simulink model "Comunicacion_Telegram_5"  (R2020b)
settings: Solver=FixedStepDiscrete  StartTime=0.0  StopTime=inf  FixedStep=0.01  RelTol=1e-3
libraries: arduinolib x15, simulink x5, pid_lib x2, commutil2 x1
settings Model: SILPILModeSetting=veronly  ExtModeTrigDuration=2  Creator=manol  LastModifiedBy=manol
settings SolverCC: AutoInsertRateTranBlk=on
settings OptimizationCC: EnhancedBackFolding=on  PassReuseOutputArgsAs=Individual arguments  ZeroExternalMemoryAtStartup=off  ZeroInternalMemoryAtStartup=off  MaxStackSize=64  OptimizeBlockOrder=speed  DifferentSizesBufferReuse=on  OptimizationCustomize=off  EfficientTunableParamExpr=on
settings DebuggingCC: ParameterTunabilityLossMsg=error
settings HardwareCC: ProdBitPerInt=16  ProdBitPerPointer=16  ProdBitPerSizeT=16  ProdBitPerPtrDiffT=16  ProdLargestAtomicFloat=None  ProdWordSize=8  ProdHWDeviceType=Atmel->AVR
settings SFSimCC: MATLABDynamicMemAlloc=off
settings RTWCC: Description=Embedded Coder  SystemTargetFile=ert.tlc  HardwareBoard=Arduino Mega 2560  TemplateMakefile=ert_default_tmf  Toolchain=Arduino AVR  BuildConfiguration=Faster Runs
settings CodeAppCC: ForceParamTrailComments=on  IgnoreCustomStorageClasses=off  OperatorAnnotations=on  SimulinkDataObjDesc=on  SFDataObjDesc=on  InsertBlockDesc=on
settings ERTTargetCC: SupportContinuousTime=on  SupportVariableSizeSignals=on  ExtModeStaticAllocSize=2048

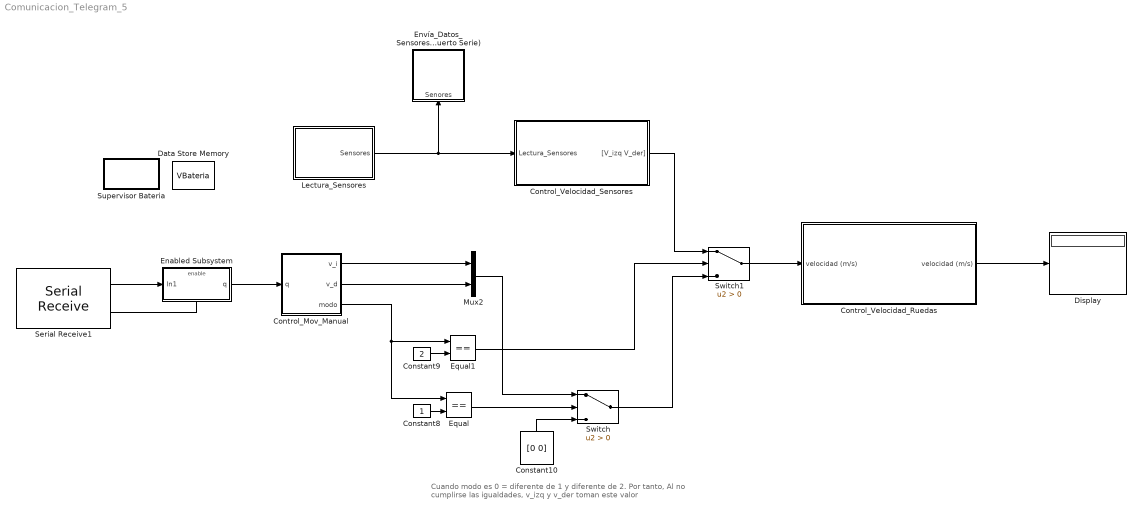
== system Comunicacion_Telegram_5 ==
  note: Cuando modo es 0 = diferente de 1 y diferente de 2.
      | Por tanto, Al no cumplirse las igualdades, v_izq y v_der toman este valor
  Constant10 : Constant  Value=[0 0]
  Constant8 : Constant
  Constant9 : Constant  Value=2
  Control_Mov_Manual : Stateflow chart  TreatAsAtomicUnit=on
  Control_Velocidad_Ruedas : Subsystem
  Control_Velocidad_Sensores : Subsystem
  Data Store Memory : DataStoreMemory  DataStoreName=VBateria  ReadBeforeWriteMsg=warning  WriteAfterWriteMsg=warning  WriteAfterReadMsg=warning  ShowAdditionalParam=off
  Display : Display
  Enabled Subsystem : Subsystem  TreatAsAtomicUnit=on
  Envía_Datos_Sensores (Puerto Serie) : Subsystem
  Equal : RelationalOperator  Operator===  OutDataTypeStr=boolean  RndMeth=Simplest
  Equal1 : RelationalOperator  Operator===  OutDataTypeStr=boolean  RndMeth=Simplest
  Lectura_Sensores : Subsystem
  Mux2 : Mux  Inputs=2
  Serial Receive1 : arduinolib/Serial Receive  isARMArch=off  portNumber=3  DataType=uint8  Datalength=1  SampleTime=0.01  showOutStatus=on  blockPlatform=arduino
      settings: SourceProductBaseCode=ARDUINO
  Supervisor Bateria : Subsystem
  Switch : Switch  Criteria=u2 > Threshold
  Switch1 : Switch  Criteria=u2 > Threshold
  wires:
  Control_Mov_Manual/3(modo) -> Equal/1, Equal1/1
  Constant10/1 -> Switch/3
  Equal1/1 -> Switch1/2
  Constant9/1 -> Equal1/2
  Switch/1 -> Switch1/3
  Serial Receive1/2 -> Enabled Subsystem/Enable
  Control_Mov_Manual/2(v_d) -> Mux2/2
  Constant8/1 -> Equal/2
  Equal/1 -> Switch/2
  Control_Mov_Manual/1(v_i) -> Mux2/1
  Enabled Subsystem/1(q) -> Control_Mov_Manual/1(q)
  Mux2/1 -> Switch/1
  Serial Receive1/1 -> Enabled Subsystem/1(In1)
  Switch1/1 -> Control_Velocidad_Ruedas/1(velocidad (m/s))
  Lectura_Sensores/1(Sensores) -> Control_Velocidad_Sensores/1(Lectura_Sensores), Envía_Datos_Sensores (Puerto Serie)/1(Senores)
  Control_Velocidad_Sensores/1("[V_izq V_der]") -> Switch1/1
  Control_Velocidad_Ruedas/1(velocidad (m/s)) -> Display/1

== system Comunicacion_Telegram_5/Control_Velocidad_Ruedas ==
  velocidad (m/s) : Inport
  Controlador (PID) : Subsystem
  Memory : Memory
  PIERO_DIY : Subsystem
  Sum : Sum  Inputs=|+-
  velocidad (m/s) : Outport  VectorParamsAs1DForOutWhenUnconnected=off
  wires:
  velocidad (m/s)/1 -> Sum/1
  PIERO_DIY/1(velocidad (m/s)) -> velocidad (m/s)/1, Memory/1
  Sum/1 -> Controlador (PID)/1(m/s)
  Controlador (PID)/1(PWM) -> PIERO_DIY/1(PWM [-255,255])
  Memory/1 -> Sum/2

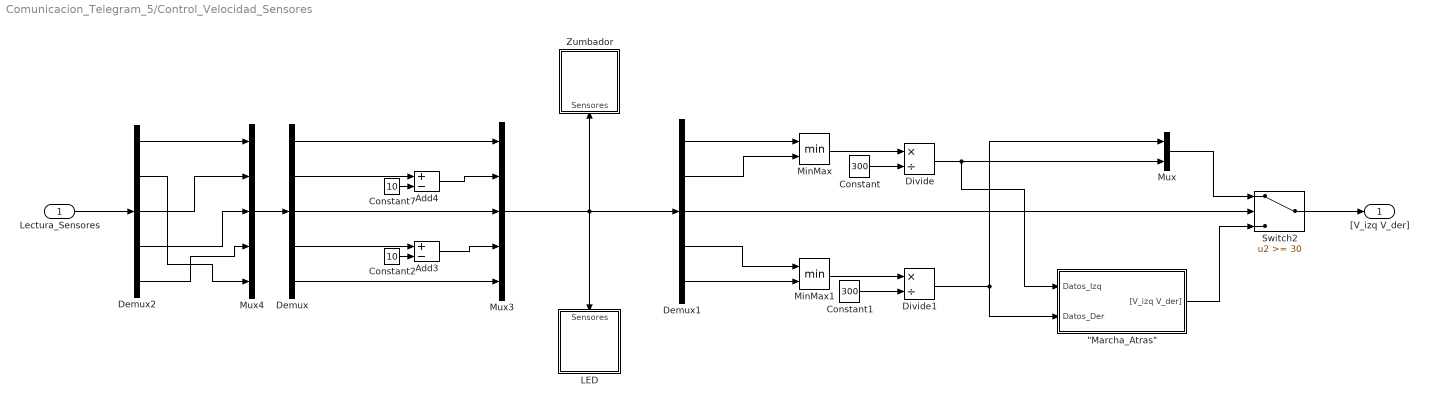
== system Comunicacion_Telegram_5/Control_Velocidad_Sensores ==
  Lectura_Sensores : Inport
  "\"Marcha_Atras\"" : Subsystem
  Add3 : Sum  Inputs=+-  AccumDataTypeStr=double  OutDataTypeStr=double
  Add4 : Sum  Inputs=+-  AccumDataTypeStr=double  OutDataTypeStr=double
  Constant : Constant  Value=300
  Constant1 : Constant  Value=300
  Constant2 : Constant  Value=10
  Constant7 : Constant  Value=10
  Demux : Demux  Outputs=5
  Demux1 : Demux  Outputs=5
  Demux2 : Demux  Outputs=5
  Divide : Product  Inputs=*/
  Divide1 : Product  Inputs=*/
  LED : Subsystem
  MinMax : MinMax  Inputs=2
  MinMax1 : MinMax  Inputs=2
  Mux : Mux  Inputs=2
  Mux3 : Mux  Inputs=5
  Mux4 : Mux  Inputs=5
  Switch2 : Switch  Threshold=30
  Zumbador : Subsystem
  "[V_izq V_der]" : Outport
  wires:
  Add3/1 -> Mux3/4
  Demux/4 -> Add3/1
  Demux1/3 -> Switch2/2
  Demux/5 -> Mux3/5
  Demux/2 -> Add4/1
  Add4/1 -> Mux3/2
  Mux3/1 -> Demux1/1, LED/1(Sensores), Zumbador/1(Sensores)
  Demux/3 -> Mux3/3
  Constant2/1 -> Add3/2
  Demux1/1 -> MinMax/1
  Constant7/1 -> Add4/2
  Demux/1 -> Mux3/1
  Constant/1 -> Divide/2
  Constant1/1 -> Divide1/2
  Divide1/1 -> "\"Marcha_Atras\""/2(Datos_Der), Mux/1
  MinMax1/1 -> Divide1/1
  Divide/1 -> "\"Marcha_Atras\""/1(Datos_Izq), Mux/2
  Demux1/2 -> MinMax/2
  Demux1/4 -> MinMax1/1
  Demux1/5 -> MinMax1/2
  Mux/1 -> Switch2/1
  Switch2/1 -> "[V_izq V_der]"/1
  MinMax/1 -> Divide/1
  "\"Marcha_Atras\""/1("[V_izq V_der]") -> Switch2/3
  Demux2/4 -> Mux4/3
  Mux4/1 -> Demux/1
  Demux2/3 -> Mux4/2
  Lectura_Sensores/1 -> Demux2/1
  Demux2/5 -> Mux4/4
  Demux2/2 -> Mux4/5
  Demux2/1 -> Mux4/1

== system Comunicacion_Telegram_5/Enabled Subsystem ==
  In1 : Inport
  Enable : EnablePort
  q : Outport
  wires:
  In1/1 -> q/1

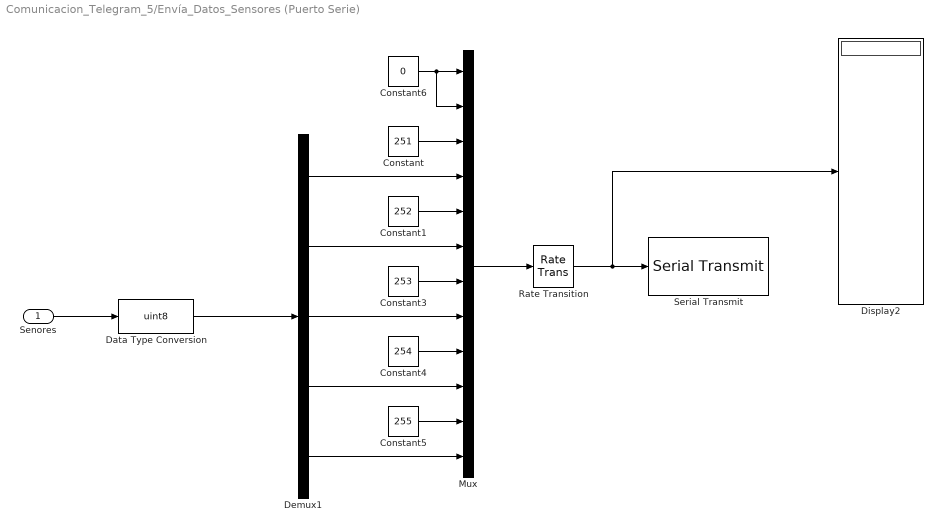
== system Comunicacion_Telegram_5/Envía_Datos_Sensores (Puerto Serie) ==
  Senores : Inport
  Constant : Constant  Value=251  OutDataTypeStr=uint8
  Constant1 : Constant  Value=252  OutDataTypeStr=uint8
  Constant3 : Constant  Value=253  OutDataTypeStr=uint8
  Constant4 : Constant  Value=254  OutDataTypeStr=uint8
  Constant5 : Constant  Value=255  OutDataTypeStr=uint8
  Constant6 : Constant  Value=0  OutDataTypeStr=uint8
  Data Type Conversion : DataTypeConversion  OutDataTypeStr=uint8
  Demux1 : Demux  Outputs=5
  Display2 : Display
  Mux : Mux  Inputs=12
  Rate Transition : RateTransition  OutPortSampleTime=1
  Serial Transmit : arduinolib/Serial Transmit  portNumber=3  sendmode=write  label=sensores  sendformat=Decimal  floatprecision=2  blockPlatform=arduino
  wires:
  Demux1/5 -> Mux/12
  Constant5/1 -> Mux/11
  Demux1/2 -> Mux/6
  Constant1/1 -> Mux/5
  Rate Transition/1 -> Display2/1, Serial Transmit/1
  Constant3/1 -> Mux/7
  Senores/1 -> Data Type Conversion/1
  Demux1/4 -> Mux/10
  Demux1/3 -> Mux/8
  Mux/1 -> Rate Transition/1
  Constant4/1 -> Mux/9
  Constant/1 -> Mux/3
  Demux1/1 -> Mux/4
  Constant6/1 -> Mux/2, Mux/1
  Data Type Conversion/1 -> Demux1/1

== system Comunicacion_Telegram_5/Lectura_Sensores ==
  LASER : Subsystem
  Mux1 : Mux  Inputs=5
  "ULTRASONIDO " : Subsystem
  Sensores : Outport
  wires:
  "ULTRASONIDO "/1(US Izquierda) -> Mux1/1
  "ULTRASONIDO "/2(US Derecha) -> Mux1/2
  LASER/1(LASER Izquierda) -> Mux1/3
  Mux1/1 -> Sensores/1
  LASER/2(LASER Centro) -> Mux1/4
  LASER/3(LASER Derecha) -> Mux1/5

== system Comunicacion_Telegram_5/Supervisor Bateria ==
  "Bateria " : arduinolib/Analog Input  pinNumber=2  ReadResultsOnly=off  ConversionTriggerSource=Software  ExternalTriggerType=uint32( 0 )  OutputDataType=uint16  EnableConversionCompleteNotify=off  EnableOuputStatus=off  SampleTime=1  blockPlatform=arduino
  Data Store Write2 : DataStoreWrite  DataStoreName=VBateria
  Gain : Gain  Gain=25/1023  OutDataTypeStr=double
  wires:
  "Bateria "/1 -> Gain/1
  Gain/1 -> Data Store Write2/1

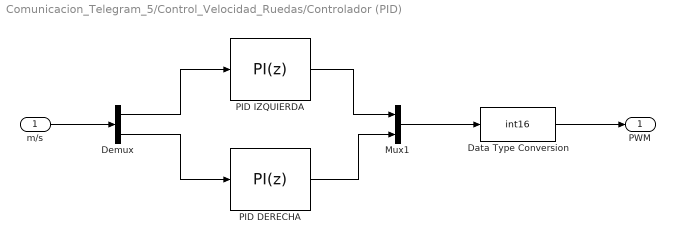
== system Comunicacion_Telegram_5/Control_Velocidad_Ruedas/Controlador (PID) ==
  m/s : Inport
  Data Type Conversion : DataTypeConversion  OutDataTypeStr=int16
  Demux : Demux  Outputs=2
  Mux1 : Mux  Inputs=2
  PID DERECHA : pid_lib/PID Controller  Controller=PI  Form=Parallel  TimeDomain=Discrete-time  UseExternalTs=off  SampleTime=0.01  IntegratorMethod=Forward Euler  FilterMethod=Forward Euler  ControllerParametersSource=internal  P=4.23623623482931  I=847.247246965862  D=0  UseFilter=on  N=100  TunerSelectOption=Transfer Function Based (PID Tuner App)  InitialConditionSource=internal  InitialConditionForIntegrator=0  InitialConditionForFilter=0  DifferentiatorICPrevScaledInput=0  ExternalReset=none  TrackingMode=off  Kt=1  LimitOutput=on  SatLimitsSource=internal  UpperSaturationLimit=255  LowerSaturationLimit=-255  LinearizeAsGain=on  AntiWindupMode=none  Kb=1  POutMin=[]  POutMax=[]  IOutMin=[]  IOutMax=[]  DOutMin=[]  DOutMax=[]  NOutMin=[]  NOutMax=[]  SumOutMin=[]  SumOutMax=[]  SaturationOutMin=[]  SaturationOutMax=[]  PParamMin=[]  PParamMax=[]  IParamMin=[]  IParamMax=[]  DParamMin=[]  DParamMax=[]  NParamMin=[]  NParamMax=[]  KbParamMin=[]  KbParamMax=[]  KtParamMin=[]  KtParamMax=[]  KbOutMin=[]  KbOutMax=[]  KtOutMin=[]  KtOutMax=[]  IntegratorOutMin=[]  IntegratorOutMax=[]  FilterOutMin=[]  FilterOutMax=[]  SumI1OutMin=[]  SumI1OutMax=[]  SumI2OutMin=[]  SumI2OutMax=[]  SumI3OutMin=[]  SumI3OutMax=[]  SumI4OutMin=[]  SumI4OutMax=[]  SumDOutMin=[]  SumDOutMax=[]  DifferentiatorOutMin=[]  DifferentiatorOutMax=[]  FilterDiffOutCoefMin=[]  FilterDiffOutCoefMax=[]  ReciprocalOutMin=[]  ReciprocalOutMax=[]  SumDenOutMin=[]  SumDenOutMax=[]  SumNumOutMin=[]  SumNumOutMax=[]  DivideOutMin=[]  DivideOutMax=[]  UdiffTsProdOutMin=[]  UdiffTsProdOutMax=[]  NTsProdOutMin=[]  NTsProdOutMax=[]  UintegralTsProdOutMin=[]  UintegralTsProdOutMax=[]  UngainTsProdOutMin=[]  UngainTsProdOutMax=[]  IntegratorContinuousStateAttributes=''  IntegratorStateMustResolveToSignalObject=off  IntegratorRTWStateStorageClass=Auto  FilterContinuousStateAttributes=''  FilterStateMustResolveToSignalObject=off  FilterRTWStateStorageClass=Auto  ParallelPVariant=InternalParameters  IdealPVariant=Disabled  IVariant=InternalParameters  DVariant=Disabled  IntegratorVariant=Discrete  SatVariant=Enabled  AWVariant=Passthrough  PCopyVariant=Disabled  TRVariant=Disabled  FdbkBlocksVariant=Forward  IdealPFdbkVariant=Disabled  SatFdbkVariant=Disabled  DerivativeFilterVariant=Disabled  NVariant=Disabled  NCopyVariant=Disabled_SignalSpec  FilterICVariant=Disabled  IntegratorICVariant=InternalICs  ExternalResetVariant=Disabled  TRSumVariant=Passthrough  SumFdbkVariant=Disabled  SumVariant=Sum_PI  TsampFilterVariant=InternalTs  TsampNgainVariant=Passthrough  TsampIntegralVariant=Passthrough  ExternalSaturationOutDataTypeStr=Inherit: Same as second input
  PID IZQUIERDA : pid_lib/PID Controller  Controller=PI  Form=Parallel  TimeDomain=Discrete-time  UseExternalTs=off  SampleTime=0.01  IntegratorMethod=Forward Euler  FilterMethod=Forward Euler  ControllerParametersSource=internal  P=4.18488568996179  I=836.977137992358  D=0  UseFilter=on  N=100  TunerSelectOption=Transfer Function Based (PID Tuner App)  InitialConditionSource=internal  InitialConditionForIntegrator=0  InitialConditionForFilter=0  DifferentiatorICPrevScaledInput=0  ExternalReset=none  TrackingMode=off  Kt=1  LimitOutput=on  SatLimitsSource=internal  UpperSaturationLimit=255  LowerSaturationLimit=-255  LinearizeAsGain=on  AntiWindupMode=none  Kb=1  POutMin=[]  POutMax=[]  IOutMin=[]  IOutMax=[]  DOutMin=[]  DOutMax=[]  NOutMin=[]  NOutMax=[]  SumOutMin=[]  SumOutMax=[]  SaturationOutMin=[]  SaturationOutMax=[]  PParamMin=[]  PParamMax=[]  IParamMin=[]  IParamMax=[]  DParamMin=[]  DParamMax=[]  NParamMin=[]  NParamMax=[]  KbParamMin=[]  KbParamMax=[]  KtParamMin=[]  KtParamMax=[]  KbOutMin=[]  KbOutMax=[]  KtOutMin=[]  KtOutMax=[]  IntegratorOutMin=[]  IntegratorOutMax=[]  FilterOutMin=[]  FilterOutMax=[]  SumI1OutMin=[]  SumI1OutMax=[]  SumI2OutMin=[]  SumI2OutMax=[]  SumI3OutMin=[]  SumI3OutMax=[]  SumI4OutMin=[]  SumI4OutMax=[]  SumDOutMin=[]  SumDOutMax=[]  DifferentiatorOutMin=[]  DifferentiatorOutMax=[]  FilterDiffOutCoefMin=[]  FilterDiffOutCoefMax=[]  ReciprocalOutMin=[]  ReciprocalOutMax=[]  SumDenOutMin=[]  SumDenOutMax=[]  SumNumOutMin=[]  SumNumOutMax=[]  DivideOutMin=[]  DivideOutMax=[]  UdiffTsProdOutMin=[]  UdiffTsProdOutMax=[]  NTsProdOutMin=[]  NTsProdOutMax=[]  UintegralTsProdOutMin=[]  UintegralTsProdOutMax=[]  UngainTsProdOutMin=[]  UngainTsProdOutMax=[]  IntegratorContinuousStateAttributes=''  IntegratorStateMustResolveToSignalObject=off  IntegratorRTWStateStorageClass=Auto  FilterContinuousStateAttributes=''  FilterStateMustResolveToSignalObject=off  FilterRTWStateStorageClass=Auto  ParallelPVariant=InternalParameters  IdealPVariant=Disabled  IVariant=InternalParameters  DVariant=Disabled  IntegratorVariant=Discrete  SatVariant=Enabled  AWVariant=Passthrough  PCopyVariant=Disabled  TRVariant=Disabled  FdbkBlocksVariant=Forward  IdealPFdbkVariant=Disabled  SatFdbkVariant=Disabled  DerivativeFilterVariant=Disabled  NVariant=Disabled  NCopyVariant=Disabled_SignalSpec  FilterICVariant=Disabled  IntegratorICVariant=InternalICs  ExternalResetVariant=Disabled  TRSumVariant=Passthrough  SumFdbkVariant=Disabled  SumVariant=Sum_PI  TsampFilterVariant=InternalTs  TsampNgainVariant=Passthrough  TsampIntegralVariant=Passthrough  ExternalSaturationOutDataTypeStr=Inherit: Same as second input
  PWM : Outport  VectorParamsAs1DForOutWhenUnconnected=off
  wires:
  Demux/1 -> PID IZQUIERDA/1
  Mux1/1 -> Data Type Conversion/1
  PID DERECHA/1 -> Mux1/2
  Demux/2 -> PID DERECHA/1
  m/s/1 -> Demux/1
  PID IZQUIERDA/1 -> Mux1/1
  Data Type Conversion/1 -> PWM/1

== system Comunicacion_Telegram_5/Control_Velocidad_Ruedas/PIERO_DIY ==
  PWM [-255,255] : Inport
  Environment Controller : simulink/Signal Routing/Environment Controller
      settings: SourceProductBaseCode=SL
  Modelo matemático PieroDIY : Subsystem
  PieroDIY-HW : Subsystem
  velocidad (m/s) : Outport  VectorParamsAs1DForOutWhenUnconnected=off
  wires:
  Environment Controller/1 -> velocidad (m/s)/1
  PWM [-255,255]/1 -> PieroDIY-HW/1(PWM 255_-255), Modelo matemático PieroDIY/1(PWM [-255,255])
  PieroDIY-HW/1(m/s) -> Environment Controller/2
  Modelo matemático PieroDIY/1(velocidad (m/s)) -> Environment Controller/1

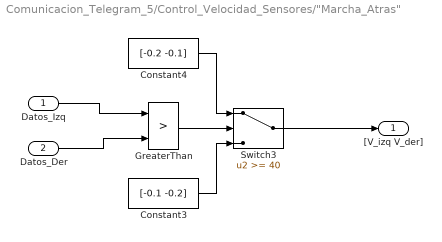
== system Comunicacion_Telegram_5/Control_Velocidad_Sensores/"Marcha_Atras" ==
  Datos_Izq : Inport
  Datos_Der : Inport  Port=2
  Constant3 : Constant  Value=[-0.1 -0.2]
  Constant4 : Constant  Value=[-0.2 -0.1]
  GreaterThan : RelationalOperator  Operator=>  OutDataTypeStr=boolean  RndMeth=Simplest
  Switch3 : Switch  Threshold=40
  "[V_izq V_der]" : Outport
  wires:
  Datos_Der/1 -> GreaterThan/2
  Constant3/1 -> Switch3/3
  Constant4/1 -> Switch3/1
  Switch3/1 -> "[V_izq V_der]"/1
  Datos_Izq/1 -> GreaterThan/1
  GreaterThan/1 -> Switch3/2

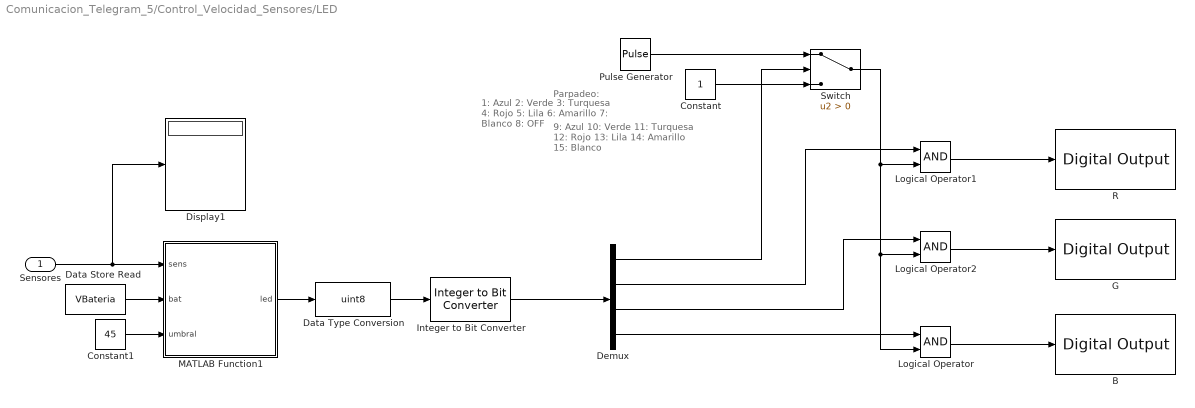
== system Comunicacion_Telegram_5/Control_Velocidad_Sensores/LED ==
  note: 9: Azul
      | 10: Verde
      | 11: Turquesa
      | 12: Rojo
      | 13: Lila
      | 14: Amarillo
      | 15: Blanco
  note: Parpadeo:
  note: 1: Azul
      | 2: Verde
      | 3: Turquesa
      | 4: Rojo
      | 5: Lila
      | 6: Amarillo
      | 7: Blanco
      | 8: OFF
  Sensores : Inport
  B : arduinolib/Digital Output  pinNumber=49  Direction=output  blockPlatform=arduino
  Constant : Constant
  Constant1 : Constant  Value=45
  Data Store Read : DataStoreRead  DataStoreName=VBateria
  Data Type Conversion : DataTypeConversion  OutDataTypeStr=uint8
  Demux : Demux
  Display1 : Display
  G : arduinolib/Digital Output  pinNumber=51  Direction=output  blockPlatform=arduino
  Integer to Bit Converter : commutil2/Integer to Bit Converter  nbits=4  signedInputValues=Unsigned  bitOrder=MSB first  outDtype=Inherit via internal rule
  Logical Operator : Logic  AllPortsSameDT=off  OutDataTypeStr=boolean
  Logical Operator1 : Logic  AllPortsSameDT=off  OutDataTypeStr=boolean
  Logical Operator2 : Logic  AllPortsSameDT=off  OutDataTypeStr=boolean
  MATLAB Function1 : MATLAB Function  TreatAsAtomicUnit=on
  Pulse Generator : DiscretePulseGenerator  PulseType=Time based  Period=0.5  PulseWidth=50
  R : arduinolib/Digital Output  pinNumber=53  Direction=output  blockPlatform=arduino
  Switch : Switch  Criteria=u2 > Threshold
  wires:
  Sensores/1 -> Display1/1, MATLAB Function1/1(sens)
  MATLAB Function1/1(led) -> Data Type Conversion/1
  Data Type Conversion/1 -> Integer to Bit Converter/1
  Integer to Bit Converter/1 -> Demux/1
  Constant/1 -> Switch/3
  Logical Operator/1 -> B/1
  Demux/2 -> Logical Operator1/1
  Logical Operator2/1 -> G/1
  Demux/3 -> Logical Operator2/1
  Demux/4 -> Logical Operator/1
  Logical Operator1/1 -> R/1
  Pulse Generator/1 -> Switch/1
  Demux/1 -> Switch/2
  Switch/1 -> Logical Operator/2, Logical Operator2/2, Logical Operator1/2
  Data Store Read/1 -> MATLAB Function1/2(bat)
  Constant1/1 -> MATLAB Function1/3(umbral)

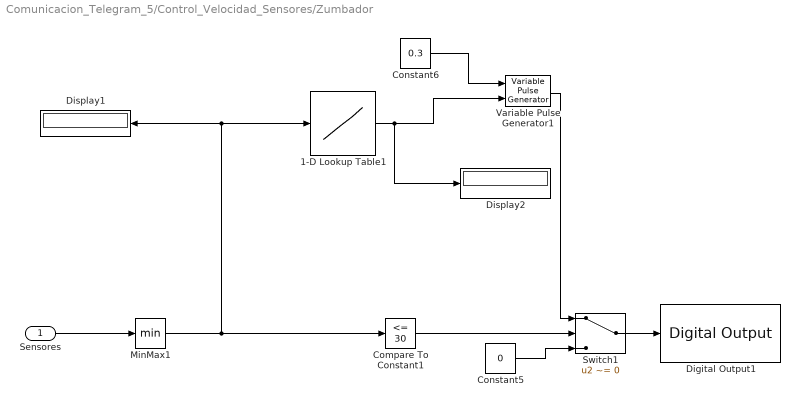
== system Comunicacion_Telegram_5/Control_Velocidad_Sensores/Zumbador ==
  Sensores : Inport
  1-D Lookup Table1 : Lookup_n-D  NumberOfTableDimensions=1  BreakpointsForDimension1=[0,9,10,19,20,29,30]  IndexSearchMethod=Linear search  Table=[0.35,0.45,0.46,0.65,0.66,0.9,0.91]  ExtrapMethod=Clip  InternalRulePriority=Speed  OutDataTypeStr=double  RndMeth=Simplest  InputSameDT=on
  Compare To Constant1 : simulink/Logic and Bit Operations/Compare To Constant  relop=<=  const=30  OutDataTypeStr=boolean
  Constant5 : Constant  Value=0
  Constant6 : Constant  Value=0.3
  Digital Output1 : arduinolib/Digital Output  pinNumber=35  Direction=output  blockPlatform=arduino
  Display1 : Display
  Display2 : Display
  MinMax1 : MinMax  OutDataTypeStr=double
  Switch1 : Switch  Criteria=u2 ~= 0
  Variable Pulse Generator1 : VariablePulseGenerator  RunAtFixedTimeIntervals=on  SampleTime=0.1
  wires:
  Variable Pulse Generator1/1 -> Switch1/1
  MinMax1/1 -> Compare To Constant1/1, 1-D Lookup Table1/1, Display1/1
  Constant6/1 -> Variable Pulse Generator1/1
  Switch1/1 -> Digital Output1/1
  Compare To Constant1/1 -> Switch1/2
  Constant5/1 -> Switch1/3
  1-D Lookup Table1/1 -> Display2/1, Variable Pulse Generator1/2
  Sensores/1 -> MinMax1/1

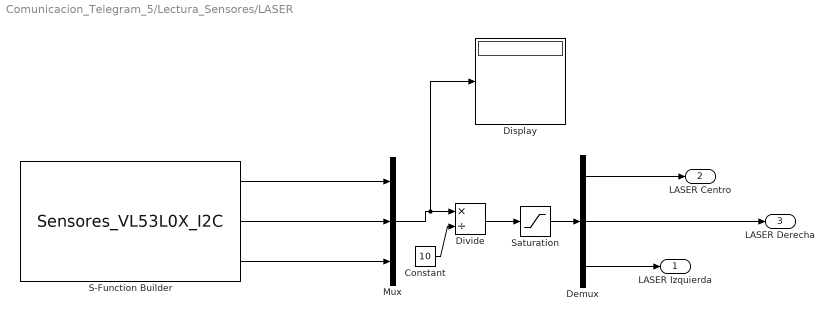
== system Comunicacion_Telegram_5/Lectura_Sensores/LASER ==
  Constant : Constant  Value=10
  Demux : Demux  Outputs=3
  Display : Display
  Divide : Product  Inputs=*/  OutDataTypeStr=int32
  Mux : Mux  Inputs=3
  S-Function Builder : S-Function  InitFcn=try, set_param(gcb,'FunctionName','Sensores_VL53L0X_I2C'), end  FunctionName=Sensores_VL53L0X_I2C  SFunctionModules=Sensores_VL53L0X_I2C_wrapper  SFunctionDeploymentMode=off  EnableBusSupport=off  mask(S-Function Builder){}
      mask help: Simulink:masks:SFunctionBuilder_MD
      mask init:
      | val = [[.9  0.75 0.75 1 1 .9 .9 1]',[1 1 0.75 0.75 .9 .9 1 .9]'];try , sys = get_param(gcb,'SfunBuilderFcnName');if isempty(sys), sys = get_param(gcb,'FunctionName'); end,catch, sys = get_param(gcb,'FunctionName'); end
      settings: CopyFcn=set_param(gcbh,'LinkStatus','none')  PreSaveFcn=try, set_param(gcb,'FunctionName','Sensores_VL53L0X_I2C'), end  OpenFcn=sfunctionwizard(gcbh)
      mask Display:
      | plot(val(:,1),val(:,2))
      | disp(sys)
      | port_label('output',1,'Sensor1')
      | port_label('output',2,'Sensor2')
      | port_label('output',3,'Sensor3')
  Saturation : Saturate  UpperLimit=255  LowerLimit=0  OutDataTypeStr=double
  LASER Izquierda : Outport  VectorParamsAs1DForOutWhenUnconnected=off
  LASER Centro : Outport  Port=2  VectorParamsAs1DForOutWhenUnconnected=off
  LASER Derecha : Outport  Port=3  VectorParamsAs1DForOutWhenUnconnected=off
  wires:
  Mux/1 -> Display/1, Divide/1
  S-Function Builder/3 -> Mux/3
  Demux/1 -> LASER Centro/1
  Demux/3 -> LASER Izquierda/1
  Divide/1 -> Saturation/1
  Saturation/1 -> Demux/1
  Constant/1 -> Divide/2
  Demux/2 -> LASER Derecha/1
  S-Function Builder/2 -> Mux/2
  S-Function Builder/1 -> Mux/1

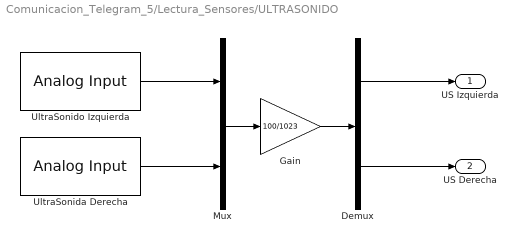
== system Comunicacion_Telegram_5/Lectura_Sensores/ULTRASONIDO  ==
  Demux : Demux  Outputs=2
  Gain : Gain  Gain=100/1023  OutDataTypeStr=double
  Mux : Mux  Inputs=2
  UltraSonida Derecha : arduinolib/Analog Input  pinNumber=0  ReadResultsOnly=off  ConversionTriggerSource=Software  ExternalTriggerType=uint32( 0 )  OutputDataType=uint16  EnableConversionCompleteNotify=off  EnableOuputStatus=off  SampleTime=0.1  blockPlatform=arduino
  UltraSonido Izquierda : arduinolib/Analog Input  pinNumber=1  ReadResultsOnly=off  ConversionTriggerSource=Software  ExternalTriggerType=uint32( 0 )  OutputDataType=uint16  EnableConversionCompleteNotify=off  EnableOuputStatus=off  SampleTime=0.1  blockPlatform=arduino
  US Izquierda : Outport
  US Derecha : Outport  Port=2
  wires:
  Demux/1 -> US Izquierda/1
  Demux/2 -> US Derecha/1
  UltraSonida Derecha/1 -> Mux/2
  UltraSonido Izquierda/1 -> Mux/1
  Mux/1 -> Gain/1
  Gain/1 -> Demux/1

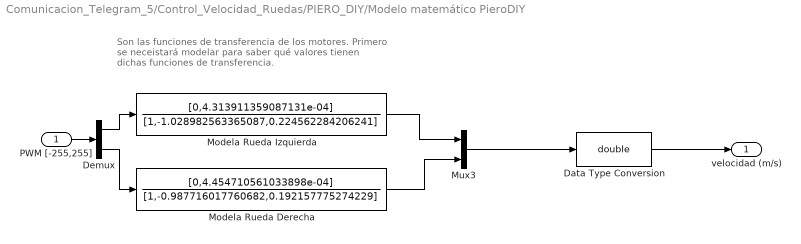
== system Comunicacion_Telegram_5/Control_Velocidad_Ruedas/PIERO_DIY/Modelo matemático PieroDIY ==
  note: Son las funciones de transferencia de los motores.
      | Primero se neceistará modelar para saber qué valores
      | tienen dichas funciones de transferencia.
  PWM [-255,255] : Inport
  Data Type Conversion : DataTypeConversion  OutDataTypeStr=double
  Demux : Demux  Outputs=2
  Modela Rueda Derecha : DiscreteFilter  Numerator=[0,4.454710561033898e-04]  Denominator=[1,-0.987716017760682,0.192157775274229]
  "Modela Rueda Izquierda " : DiscreteFilter  Numerator=[0,4.313911359087131e-04]  Denominator=[1,-1.028982563365087,0.224562284206241]
  Mux3 : Mux  Inputs=2
  velocidad (m/s) : Outport  VectorParamsAs1DForOutWhenUnconnected=off
  wires:
  Demux/2 -> Modela Rueda Derecha/1
  Data Type Conversion/1 -> velocidad (m/s)/1
  Demux/1 -> "Modela Rueda Izquierda "/1
  Mux3/1 -> Data Type Conversion/1
  Modela Rueda Derecha/1 -> Mux3/2
  PWM [-255,255]/1 -> Demux/1
  "Modela Rueda Izquierda "/1 -> Mux3/1

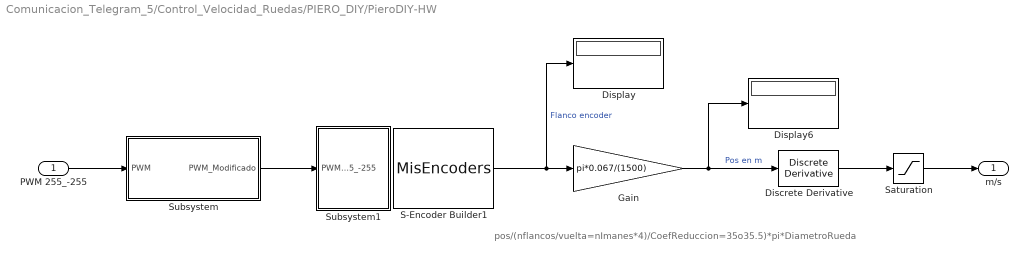
== system Comunicacion_Telegram_5/Control_Velocidad_Ruedas/PIERO_DIY/PieroDIY-HW ==
  note: pos/(nflancos/vuelta=nImanes*4)/CoefReduccion=35o35.5)*pi*DiametroRueda
  PWM 255_-255 : Inport
  Discrete Derivative : simulink/Discrete/Discrete Derivative  gainval=1.0  ICPrevScaledInput=0.0  OutMin=[]  OutMax=[]  OutDataTypeStr=double  OutputDataTypeScalingMode=double  OutDataType=fixdt(1, 16)  OutScaling=2^-10  DoSatur=off
  Display : Display
  Display6 : Display
  Gain : Gain  Gain=pi*0.067/(1500)  OutDataTypeStr=double
  S-Encoder Builder1 : S-Function  FunctionName=MisEncoders  Parameters=uint8(18),uint8(19),int8(1),uint8(2),uint8(3),uint8(0)  SFunctionModules=MisEncoders_wrapper  SFunctionDeploymentMode=off  EnableBusSupport=off  mask(S-Function Builder){}
      mask help: Simulink:masks:SFunctionBuilder_MD
      mask init: same as Comunicacion_Telegram_5/Lectura_Sensores/LASER/S-Function Builder
      settings: CopyFcn=set_param(gcbh,'LinkStatus','none')  PreSaveFcn=try, set_param(gcb,'FunctionName','MisEncoders'), end  OpenFcn=sfunctionwizard(gcbh)
      mask Display:
      | plot(val(:,1),val(:,2))
      | disp(sys)
      | port_label('output',1,'pos')
  Saturation : Saturate  UpperLimit=0.6  LowerLimit=-0.6  OutDataTypeStr=double
  Subsystem : Subsystem
  Subsystem1 : Subsystem
  m/s : Outport  VectorParamsAs1DForOutWhenUnconnected=off
  wires:
  Discrete Derivative/1 -> Saturation/1
  Saturation/1 -> m/s/1
  Gain/1 -> Display6/1, Discrete Derivative/1  "Pos en m"
  S-Encoder Builder1/1 -> Display/1, Gain/1  "Flanco encoder"
  PWM 255_-255/1 -> Subsystem/1(PWM)
  Subsystem/1(PWM_Modificado) -> Subsystem1/1(PWM 255_-255)

== system Comunicacion_Telegram_5/Control_Velocidad_Ruedas/PIERO_DIY/PieroDIY-HW/Subsystem ==
  PWM : Inport
  Constant : Constant  Value=12.2
  Data Store Read : DataStoreRead  DataStoreName=VBateria
  Divide : Product  Inputs=*/
  Divide1 : Product  Inputs=*/
  PWM_Modificado : Outport
  wires:
  Constant/1 -> Divide1/2
  Divide1/1 -> Divide/2
  Data Store Read/1 -> Divide1/1
  PWM/1 -> Divide/1
  Divide/1 -> PWM_Modificado/1

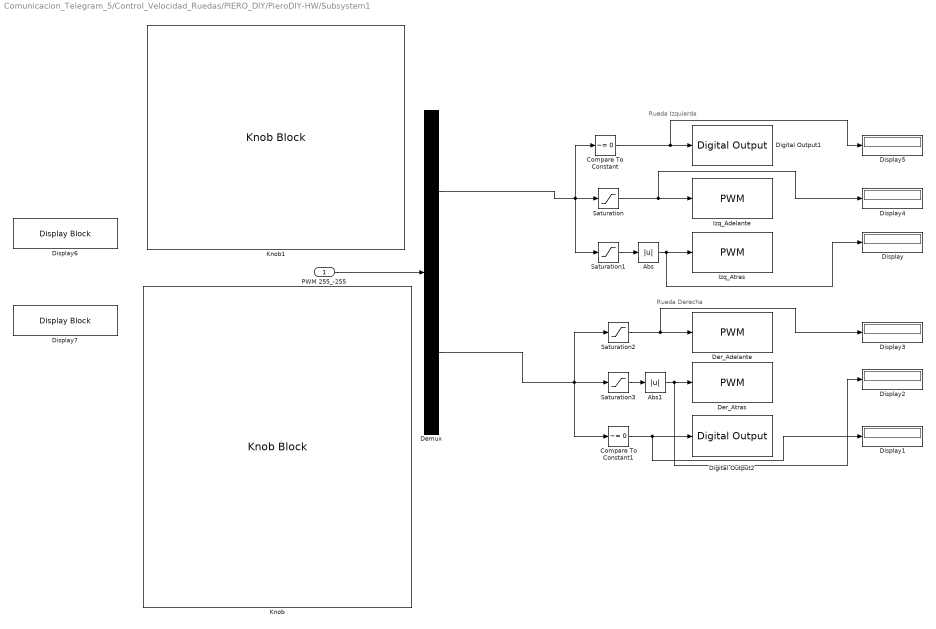
== system Comunicacion_Telegram_5/Control_Velocidad_Ruedas/PIERO_DIY/PieroDIY-HW/Subsystem1 ==
  note: Rueda Derecha
  note: Rueda Izquierda
  PWM 255_-255 : Inport
  Abs : Abs  OutDataTypeStr=uint8
  Abs1 : Abs  OutDataTypeStr=uint8
  Compare To Constant : simulink/Logic and Bit Operations/Compare To Constant  relop=~=  const=0  OutDataTypeStr=boolean
  Compare To Constant1 : simulink/Logic and Bit Operations/Compare To Constant  relop=~=  const=0  OutDataTypeStr=boolean
  Demux : Demux  Outputs=2
  Der_Adelante : arduinolib/PWM  pinNumber=8  frequencyType=Default  desiredFrequency=490.2  achievableFrequency=490.2
  Der_Atras : arduinolib/PWM  pinNumber=9  frequencyType=Default  desiredFrequency=490.2  achievableFrequency=490.2
  Digital Output1 : arduinolib/Digital Output  pinNumber=5  Direction=output  blockPlatform=arduino
  Digital Output2 : arduinolib/Digital Output  pinNumber=10  Direction=output  blockPlatform=arduino
  Display{,1..5} (6 alike) : Display
  Display6 : DisplayBlock  LabelPosition=Hide
  Display7 : DisplayBlock  LabelPosition=Hide
  Izq_Adelante : arduinolib/PWM  pinNumber=6  frequencyType=Default  desiredFrequency=490.2  achievableFrequency=490.2
  Izq_Atras : arduinolib/PWM  pinNumber=7  frequencyType=Default  desiredFrequency=490.2  achievableFrequency=490.2
  Knob : KnobBlock
  Knob1 : KnobBlock
  Saturation : Saturate  UpperLimit=255  LowerLimit=0
  Saturation1 : Saturate  UpperLimit=0  LowerLimit=-255
  Saturation2 : Saturate  UpperLimit=255  LowerLimit=0
  Saturation3 : Saturate  UpperLimit=0  LowerLimit=-255
  wires:
  Saturation/1 -> Display4/1, Izq_Adelante/1
  Compare To Constant/1 -> Display5/1, Digital Output1/1
  Saturation1/1 -> Abs/1
  PWM 255_-255/1 -> Demux/1
  Demux/1 -> Saturation1/1, Compare To Constant/1, Saturation/1
  Abs/1 -> Display/1, Izq_Atras/1
  Saturation3/1 -> Abs1/1
  Demux/2 -> Compare To Constant1/1, Saturation2/1, Saturation3/1
  Compare To Constant1/1 -> Display1/1, Digital Output2/1
  Abs1/1 -> Display2/1, Der_Atras/1
  Saturation2/1 -> Display3/1, Der_Adelante/1

== matlab function Comunicacion_Telegram_5/Control_Velocidad_Sensores/LED/MATLAB Function1 ==
  data: sens input; led output; bat input; umbral input
function led  = fcn(sens, bat, umbral)


led  = 2; %Verde

if (bat <= 11.2)
    led = 12; %Rojo + Parp
else
    
    if (sens(3) <= umbral)
        led = 15; %Blanco + Parp
    else
        if (sens(1) <= umbral && sens(2) <= umbral)
            led = 1; %Azul
        else
            if (sens(1) <= umbral)
                led = 3; %Turquesa
            end
            if (sens(2) <= umbral)
                led = 11; %Turquesa + Parp.
            end
        end
        if (sens(4) <= umbral && sens(5) <= umbral)
            led = 6; %Amarillo
        else
            if (sens(4) <= umbral) 
                led = 13; %Lila + Parp.
            end
            if (sens(5) <= umbral)
                led = 5; %Lila
            end
        end
    end
end

== stateflow chart Comunicacion_Telegram_5/Control_Mov_Manual ==
  state nada
    v_i=0;
    v_d=0;
    modo=0;
  state espera1
  state Evita_obs
    entry:
    modo=2;
  state Primera_etiqueta_X1
  state espera
    entry:
    modo=1;
  state Derecha
    entry:
    if(v_d<=0.4 & v_d>=-0.2)
    v_i=v_i+0.05;
    v_d=v_d-0.02;
    end;
  state Izquierda
    entry:
    if(v_i<=0.4 & v_d>=-0.2)
    v_d=v_d+0.05;
    v_i=v_i-0.02;
    end;
  state Primera_etiqueta_X
  state Atras
    entry:
    if(v_d>=-0.2 & v_i>=-0.2)
    v_d=v_d-0.05;
    v_i=v_i-0.05;
    end;
  state Adelante
    entry:
    if(v_i<=0.4 & v_d<=0.4)
    v_i=v_i+0.05;
    v_d=v_d+0.05;
    end;
  state Parar
    entry:
    v_i=0;
    v_d=0;
  (default) -> nada
  Primera_etiqueta_X -> nada [order 2] : [q==82]
  Primera_etiqueta_X1 -> nada [order 3] : [q==82]
  nada -> espera1
  espera1 -> Primera_etiqueta_X1 : [q==88]
  Primera_etiqueta_X1 -> Evita_obs [order 2] : [q==69]
  Evita_obs -> Primera_etiqueta_X1 : [q==88]
  Primera_etiqueta_X1 -> espera [order 1] : [q==77]
  Derecha -> espera
  Izquierda -> espera
  Parar -> espera
  Atras -> espera
  Adelante -> espera
  Primera_etiqueta_X -> espera [order 7] : [q==77]
  espera -> Primera_etiqueta_X : [q==88]
  Primera_etiqueta_X -> Derecha [order 3] : [q==68]
  Primera_etiqueta_X -> Izquierda [order 1] : [q==65]
  Primera_etiqueta_X -> Atras [order 5] : [q==83]
  Primera_etiqueta_X -> Adelante [order 4] : [q==87]
  Primera_etiqueta_X -> Parar [order 6] : [q==32]
  data: v_i output; q input; v_d output; modo output
